simulink model "LiftModel"  (R2020a)
settings: Solver=VariableStepAuto  StartTime=0.0  StopTime=10.0  RelTol=1e-3
libraries: simulink_extras x1
settings Model: Creator=Admin  LastModifiedBy=Admin

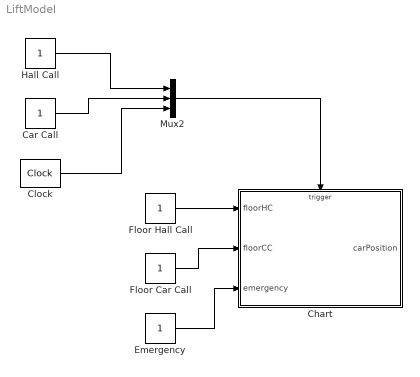
== system LiftModel ==
  Car Call : Constant
  Chart : Stateflow chart  TreatAsAtomicUnit=on
  Clock : simulink_extras/Flip Flops/Clock  period=2
  Emergency : Constant
  Floor Car Call : Constant
  "Floor Hall Call " : Constant
  Hall Call : Constant
  Mux2 : Mux  Inputs=3
  wires:
  Hall Call/1 -> Mux2/1
  Car Call/1 -> Mux2/2
  Mux2/1 -> Chart/Trigger
  Clock/1 -> Mux2/3
  Floor Car Call/1 -> Chart/2(floorCC)
  "Floor Hall Call "/1 -> Chart/1(floorHC)
  Emergency/1 -> Chart/3(emergency)

== stateflow chart LiftModel/Chart ==
  state STATUS
    state BUSY
    state IDLE
    (default) -> IDLE
    IDLE -> BUSY
  (default) -> STATUS
  data: carPosition output; floorHC input; floorCC input; emergency input
  events: CC input RISING_EDGE_EVENT; HC input RISING_EDGE_EVENT; clock input RISING_EDGE_EVENT
